simulink model "cst_robotarm_breach"  (R2020a)
settings: Solver=ode23t  StartTime=0.0  StopTime=40  FixedStep=0.0001  MaxStep=0.05  RelTol=1e-3  EnableMultiTasking=on
model workspace (MAT data in the model file):
  DCMotor_J = 0.0946866703633
  DCMotor_K = 0.477771340295
  DCMotor_Kf = 0.921434142151
  DCMotor_L = 0.000316454712175
  DCMotor_R = 4.99938152603
  Ts = 0.1
  dFilt = [1 -0.1202]
  nFilt = [0.4399 0.4399]
undefined symbols (not defined in the file or in its folder): X, Y, Z
libraries: sm_lib x244, fl_lib x75, nesl_utility x28, ee_lib x21
(part 5 of 6)

== system cst_robotarm_breach/6 DOF Robot Arm/6 DOF Robot Arm Mechanics/Forearm/ServoTJD_2_RIGID/servo_cover_2_RIGID ==
  ReferenceFrame : sm_lib/Frames and Transforms/Reference Frame
  Solid : sm_lib/Body Elements/File Solid  ExtGeomFileName=servo cover_Default_sldprt.STL  UnitType=Custom  ExtGeomFileUnits=mm  StepReaderType=HEX  ExportConvexHullGeometry=off  InertiaType=Custom  Mass=0.018198073455255783  MassUnits=kg  CenterOfMass=[19.173079671185903 9.8425000000000011 6.6069555093490839]  CenterOfMassUnits=mm  MomentsOfInertia=[1.0514460019053871 4.1870037592553642 4.7863110501402781]  MomentsOfInertiaUnits=kg*mm^2  ProductsOfInertia=[0 0.046415809435786888 0]  ProductsOfInertiaUnits=kg*mm^2  BasedOnType=Density  Density=1000  DensityUnits=kg/(m^3)  DoExposeReferenceFrame=on  SerializedFrames=<Frames/>  GraphicType=FromGeometry  MarkerShape=Sphere  MarkerSize=10  MarkerSizeUnits=m  GraphicVisPropType=SimpleVisualProperties  GraphicDiffuseColor=[0.6 0.6 0.6]  GraphicSpecularColor=[0.5 0.5 0.5 1.0]  GraphicAmbientColor=[0.15 0.15 0.15 1.0]  GraphicEmissiveColor=[0.0 0.0 0.0 1.0]  GraphicShininess=75  GraphicOpacity=1
  F : PMIOPort  Side=Left
  connections:
  Solid/RConn1 -- ReferenceFrame/RConn1 -- F/RConn1

== system cst_robotarm_breach/6 DOF Robot Arm/6 DOF Robot Arm Mechanics/Forearm/UpperArm_1_RIGID/BaseRef_1_RIGID ==
  ReferenceFrame : sm_lib/Frames and Transforms/Reference Frame
  Solid : sm_lib/Body Elements/File Solid  ExtGeomFileName=BaseRef_Default_sldprt.STL  UnitType=Custom  ExtGeomFileUnits=in  StepReaderType=HEX  ExportConvexHullGeometry=off  InertiaType=Custom  Mass=0.0048917083782427382  MassUnits=kg  CenterOfMass=[-1.7039170891361811e-10 0.2623949674376988 1.6125651751179532e-08]  CenterOfMassUnits=in  MomentsOfInertia=[0.0003243123013680548 0.00029766954875355879 0.00032242565061571212]  MomentsOfInertiaUnits=kg*in^2  ProductsOfInertia=[-6.4526471956204744e-12 2.3575705931561807e-11 0]  ProductsOfInertiaUnits=kg*in^2  BasedOnType=Density  Density=1000  DensityUnits=kg/(m^3)  DoExposeReferenceFrame=on  SerializedFrames=<Frames/>  GraphicType=FromGeometry  MarkerShape=Sphere  MarkerSize=10  MarkerSizeUnits=m  GraphicVisPropType=SimpleVisualProperties  GraphicDiffuseColor=[0.6 0.8 1.0]  GraphicSpecularColor=[0.5 0.5 0.5 1.0]  GraphicAmbientColor=[0.15 0.15 0.15 1.0]  GraphicEmissiveColor=[0.0 0.0 0.0 1.0]  GraphicShininess=75  GraphicOpacity=1
  F : PMIOPort  Side=Left
  connections:
  Solid/RConn1 -- ReferenceFrame/RConn1 -- F/RConn1

== system cst_robotarm_breach/6 DOF Robot Arm/6 DOF Robot Arm Mechanics/Forearm/UpperArm_1_RIGID/BaseRef_2_RIGID ==
  ReferenceFrame : sm_lib/Frames and Transforms/Reference Frame
  Solid : sm_lib/Body Elements/File Solid  ExtGeomFileName=BaseRef_Default_sldprt.STL  UnitType=Custom  ExtGeomFileUnits=in  StepReaderType=HEX  ExportConvexHullGeometry=off  InertiaType=Custom  Mass=0.0048917083782427382  MassUnits=kg  CenterOfMass=[-1.7039170891361811e-10 0.2623949674376988 1.6125651751179532e-08]  CenterOfMassUnits=in  MomentsOfInertia=[0.0003243123013680548 0.00029766954875355879 0.00032242565061571212]  MomentsOfInertiaUnits=kg*in^2  ProductsOfInertia=[-6.4526471956204744e-12 2.3575705931561807e-11 0]  ProductsOfInertiaUnits=kg*in^2  BasedOnType=Density  Density=1000  DensityUnits=kg/(m^3)  DoExposeReferenceFrame=on  SerializedFrames=<Frames/>  GraphicType=FromGeometry  MarkerShape=Sphere  MarkerSize=10  MarkerSizeUnits=m  GraphicVisPropType=SimpleVisualProperties  GraphicDiffuseColor=[0.6 0.8 1.0]  GraphicSpecularColor=[0.5 0.5 0.5 1.0]  GraphicAmbientColor=[0.15 0.15 0.15 1.0]  GraphicEmissiveColor=[0.0 0.0 0.0 1.0]  GraphicShininess=75  GraphicOpacity=1
  F : PMIOPort  Side=Left
  connections:
  Solid/RConn1 -- ReferenceFrame/RConn1 -- F/RConn1

== system cst_robotarm_breach/6 DOF Robot Arm/6 DOF Robot Arm Mechanics/Forearm/UpperArm_1_RIGID/asb_04_1_RIGID ==
  ReferenceFrame : sm_lib/Frames and Transforms/Reference Frame
  Solid : sm_lib/Body Elements/File Solid  ExtGeomFileName=asb-04_Default_sldprt.STL  UnitType=Custom  ExtGeomFileUnits=mm  StepReaderType=HEX  ExportConvexHullGeometry=off  InertiaType=Custom  Mass=0.012502145661798053  MassUnits=kg  CenterOfMass=[0 6.0244491918420078 4.4962453719208186]  CenterOfMassUnits=mm  MomentsOfInertia=[2.428586923331026 4.8465793426778037 3.7918219462476519]  MomentsOfInertiaUnits=kg*mm^2  ProductsOfInertia=[-0.330066861743673 0 0]  ProductsOfInertiaUnits=kg*mm^2  BasedOnType=Density  Density=1000  DensityUnits=kg/(m^3)  DoExposeReferenceFrame=on  SerializedFrames=<Frames/>  GraphicType=FromGeometry  MarkerShape=Sphere  MarkerSize=10  MarkerSizeUnits=m  GraphicVisPropType=SimpleVisualProperties  GraphicDiffuseColor=[0.6 0.8 1.0]  GraphicSpecularColor=[0.5 0.5 0.5 1.0]  GraphicAmbientColor=[0.15 0.15 0.15 1.0]  GraphicEmissiveColor=[0.0 0.0 0.0 1.0]  GraphicShininess=75  GraphicOpacity=1
  F : PMIOPort  Side=Left
  connections:
  Solid/RConn1 -- ReferenceFrame/RConn1 -- F/RConn1

== system cst_robotarm_breach/6 DOF Robot Arm/6 DOF Robot Arm Mechanics/Forearm/UpperArm_1_RIGID/asb_04_2_RIGID ==
  ReferenceFrame : sm_lib/Frames and Transforms/Reference Frame
  Solid : sm_lib/Body Elements/File Solid  ExtGeomFileName=asb-04_Default_sldprt.STL  UnitType=Custom  ExtGeomFileUnits=mm  StepReaderType=HEX  ExportConvexHullGeometry=off  InertiaType=Custom  Mass=0.012502145661798053  MassUnits=kg  CenterOfMass=[0 6.0244491918420078 4.4962453719208186]  CenterOfMassUnits=mm  MomentsOfInertia=[2.428586923331026 4.8465793426778037 3.7918219462476519]  MomentsOfInertiaUnits=kg*mm^2  ProductsOfInertia=[-0.330066861743673 0 0]  ProductsOfInertiaUnits=kg*mm^2  BasedOnType=Density  Density=1000  DensityUnits=kg/(m^3)  DoExposeReferenceFrame=on  SerializedFrames=<Frames/>  GraphicType=FromGeometry  MarkerShape=Sphere  MarkerSize=10  MarkerSizeUnits=m  GraphicVisPropType=SimpleVisualProperties  GraphicDiffuseColor=[0.6 0.8 1.0]  GraphicSpecularColor=[0.5 0.5 0.5 1.0]  GraphicAmbientColor=[0.15 0.15 0.15 1.0]  GraphicEmissiveColor=[0.0 0.0 0.0 1.0]  GraphicShininess=75  GraphicOpacity=1
  F : PMIOPort  Side=Left
  connections:
  Solid/RConn1 -- ReferenceFrame/RConn1 -- F/RConn1

== system cst_robotarm_breach/6 DOF Robot Arm/6 DOF Robot Arm Mechanics/Forearm/UpperArm_1_RIGID/asb_06_1_RIGID ==
  ReferenceFrame : sm_lib/Frames and Transforms/Reference Frame
  Solid : sm_lib/Body Elements/File Solid  ExtGeomFileName=asb-06_Default_sldprt.STL  UnitType=Custom  ExtGeomFileUnits=mm  StepReaderType=HEX  ExportConvexHullGeometry=off  InertiaType=Custom  Mass=0.0080717858989095559  MassUnits=kg  CenterOfMass=[-9.9260131397596147 6.2234969189440275 0]  CenterOfMassUnits=mm  MomentsOfInertia=[0.871366295206629 1.2650443449488296 1.3334610494978376]  MomentsOfInertiaUnits=kg*mm^2  ProductsOfInertia=[0 0 -0.36019818264401821]  ProductsOfInertiaUnits=kg*mm^2  BasedOnType=Density  Density=1000  DensityUnits=kg/(m^3)  DoExposeReferenceFrame=on  SerializedFrames=<Frames/>  GraphicType=FromGeometry  MarkerShape=Sphere  MarkerSize=10  MarkerSizeUnits=m  GraphicVisPropType=SimpleVisualProperties  GraphicDiffuseColor=[0.6 0.8 1.0]  GraphicSpecularColor=[0.5 0.5 0.5 1.0]  GraphicAmbientColor=[0.15 0.15 0.15 1.0]  GraphicEmissiveColor=[0.0 0.0 0.0 1.0]  GraphicShininess=75  GraphicOpacity=1
  F : PMIOPort  Side=Left
  connections:
  Solid/RConn1 -- ReferenceFrame/RConn1 -- F/RConn1

== system cst_robotarm_breach/6 DOF Robot Arm/6 DOF Robot Arm Mechanics/Forearm/UpperArm_1_RIGID/asb_06_2_RIGID ==
  ReferenceFrame : sm_lib/Frames and Transforms/Reference Frame
  Solid : sm_lib/Body Elements/File Solid  ExtGeomFileName=asb-06_Default_sldprt.STL  UnitType=Custom  ExtGeomFileUnits=mm  StepReaderType=HEX  ExportConvexHullGeometry=off  InertiaType=Custom  Mass=0.0080717858989095559  MassUnits=kg  CenterOfMass=[-9.9260131397596147 6.2234969189440275 0]  CenterOfMassUnits=mm  MomentsOfInertia=[0.871366295206629 1.2650443449488296 1.3334610494978376]  MomentsOfInertiaUnits=kg*mm^2  ProductsOfInertia=[0 0 -0.36019818264401821]  ProductsOfInertiaUnits=kg*mm^2  BasedOnType=Density  Density=1000  DensityUnits=kg/(m^3)  DoExposeReferenceFrame=on  SerializedFrames=<Frames/>  GraphicType=FromGeometry  MarkerShape=Sphere  MarkerSize=10  MarkerSizeUnits=m  GraphicVisPropType=SimpleVisualProperties  GraphicDiffuseColor=[0.6 0.8 1.0]  GraphicSpecularColor=[0.5 0.5 0.5 1.0]  GraphicAmbientColor=[0.15 0.15 0.15 1.0]  GraphicEmissiveColor=[0.0 0.0 0.0 1.0]  GraphicShininess=75  GraphicOpacity=1
  F : PMIOPort  Side=Left
  connections:
  Solid/RConn1 -- ReferenceFrame/RConn1 -- F/RConn1

== system cst_robotarm_breach/6 DOF Robot Arm/6 DOF Robot Arm Mechanics/Forearm/UpperArm_1_RIGID/at_06_1_RIGID ==
  ReferenceFrame : sm_lib/Frames and Transforms/Reference Frame
  Solid : sm_lib/Body Elements/File Solid  ExtGeomFileName=at-06_Default_sldprt.STL  UnitType=Custom  ExtGeomFileUnits=mm  StepReaderType=HEX  ExportConvexHullGeometry=off  InertiaType=Custom  Mass=0.0081837500372110746  MassUnits=kg  CenterOfMass=[-1.816422467996463e-08 -5.0466522298709023e-07 42.862382459231029]  CenterOfMassUnits=mm  MomentsOfInertia=[5.0863463702079237 5.0907330809753244 0.28704603607760404]  MomentsOfInertiaUnits=kg*mm^2  ProductsOfInertia=[2.9075703783527806e-06 -7.690574725829705e-07 -3.4008607477439507e-06]  ProductsOfInertiaUnits=kg*mm^2  BasedOnType=Density  Density=1000  DensityUnits=kg/(m^3)  DoExposeReferenceFrame=on  SerializedFrames=<Frames/>  GraphicType=FromGeometry  MarkerShape=Sphere  MarkerSize=10  MarkerSizeUnits=m  GraphicVisPropType=SimpleVisualProperties  GraphicDiffuseColor=[0.6 0.8 1.0]  GraphicSpecularColor=[0.5 0.5 0.5 1.0]  GraphicAmbientColor=[0.15 0.15 0.15 1.0]  GraphicEmissiveColor=[0.0 0.0 0.0 1.0]  GraphicShininess=75  GraphicOpacity=1
  F : PMIOPort  Side=Left
  connections:
  Solid/RConn1 -- ReferenceFrame/RConn1 -- F/RConn1

== system cst_robotarm_breach/6 DOF Robot Arm/6 DOF Robot Arm Mechanics/Gripper/LeftGripper_1_RIGID/GripperLeft_1_RIGID ==
  ReferenceFrame : sm_lib/Frames and Transforms/Reference Frame
  Solid : sm_lib/Body Elements/File Solid  ExtGeomFileName=GripperLeft_Default_sldprt.STL  UnitType=Custom  ExtGeomFileUnits=mm  StepReaderType=HEX  ExportConvexHullGeometry=off  InertiaType=Custom  Mass=0.0054837472367652322  MassUnits=kg  CenterOfMass=[7.5312895024124931 -5.3079249665701553 1.2060569262790406]  CenterOfMassUnits=mm  MomentsOfInertia=[0.28663713454900869 0.89920807040371731 0.71744303970434065]  MomentsOfInertiaUnits=kg*mm^2  ProductsOfInertia=[-0.013166116487360812 0.10888352596311582 0.088149803089705936]  ProductsOfInertiaUnits=kg*mm^2  BasedOnType=Density  Density=1000  DensityUnits=kg/(m^3)  DoExposeReferenceFrame=on  SerializedFrames=<Frames/>  GraphicType=FromGeometry  MarkerShape=Sphere  MarkerSize=10  MarkerSizeUnits=m  GraphicVisPropType=SimpleVisualProperties  GraphicDiffuseColor=[0.4 0.4 0.4]  GraphicSpecularColor=[0.5 0.5 0.5 1.0]  GraphicAmbientColor=[0.15 0.15 0.15 1.0]  GraphicEmissiveColor=[0.0 0.0 0.0 1.0]  GraphicShininess=75  GraphicOpacity=1
  F : PMIOPort  Side=Left
  connections:
  Solid/RConn1 -- ReferenceFrame/RConn1 -- F/RConn1

== system cst_robotarm_breach/6 DOF Robot Arm/6 DOF Robot Arm Mechanics/Gripper/LeftGripper_1_RIGID/gripperPad_1_RIGID ==
  ReferenceFrame : sm_lib/Frames and Transforms/Reference Frame
  Solid : sm_lib/Body Elements/File Solid  ExtGeomFileName=gripperPad_Default_sldprt.STL  UnitType=Custom  ExtGeomFileUnits=mm  StepReaderType=HEX  ExportConvexHullGeometry=off  InertiaType=Custom  Mass=0.0014400000000000001  MassUnits=kg  CenterOfMass=[0 0 0]  CenterOfMassUnits=mm  MomentsOfInertia=[0.040799999999999996 0.049920000000000006 0.086880000000000027]  MomentsOfInertiaUnits=kg*mm^2  ProductsOfInertia=[0 0 0]  ProductsOfInertiaUnits=kg*mm^2  BasedOnType=Density  Density=1000  DensityUnits=kg/(m^3)  DoExposeReferenceFrame=on  SerializedFrames=<Frames/>  GraphicType=FromGeometry  MarkerShape=Sphere  MarkerSize=10  MarkerSizeUnits=m  GraphicVisPropType=SimpleVisualProperties  GraphicDiffuseColor=[0.3 0.3 0.3]  GraphicSpecularColor=[0.5 0.5 0.5 1.0]  GraphicAmbientColor=[0.15 0.15 0.15 1.0]  GraphicEmissiveColor=[0.0 0.0 0.0 1.0]  GraphicShininess=75  GraphicOpacity=1
  F : PMIOPort  Side=Left
  connections:
  Solid/RConn1 -- ReferenceFrame/RConn1 -- F/RConn1

== system cst_robotarm_breach/6 DOF Robot Arm/6 DOF Robot Arm Mechanics/Gripper/RightGripper_1_RIGID/GripperRight_1_RIGID ==
  ReferenceFrame : sm_lib/Frames and Transforms/Reference Frame
  Solid : sm_lib/Body Elements/File Solid  ExtGeomFileName=GripperRight_Default_sldprt.STL  UnitType=Custom  ExtGeomFileUnits=mm  StepReaderType=HEX  ExportConvexHullGeometry=off  InertiaType=Custom  Mass=0.0054837472367652304  MassUnits=kg  CenterOfMass=[7.5312895024124948 -5.3079249665701571 -1.2060569262790404]  CenterOfMassUnits=mm  MomentsOfInertia=[0.28663713454900847 0.8992080704037172 0.71744303970434065]  MomentsOfInertiaUnits=kg*mm^2  ProductsOfInertia=[0.013166116487360839 -0.10888352596311589 0.088149803089706033]  ProductsOfInertiaUnits=kg*mm^2  BasedOnType=Density  Density=1000  DensityUnits=kg/(m^3)  DoExposeReferenceFrame=on  SerializedFrames=<Frames/>  GraphicType=FromGeometry  MarkerShape=Sphere  MarkerSize=10  MarkerSizeUnits=m  GraphicVisPropType=SimpleVisualProperties  GraphicDiffuseColor=[0.4 0.4 0.4]  GraphicSpecularColor=[0.5 0.5 0.5 1.0]  GraphicAmbientColor=[0.15 0.15 0.15 1.0]  GraphicEmissiveColor=[0.0 0.0 0.0 1.0]  GraphicShininess=75  GraphicOpacity=1
  F : PMIOPort  Side=Left
  connections:
  Solid/RConn1 -- ReferenceFrame/RConn1 -- F/RConn1

== system cst_robotarm_breach/6 DOF Robot Arm/6 DOF Robot Arm Mechanics/Gripper/RightGripper_1_RIGID/gripperPad_1_RIGID ==
  ReferenceFrame : sm_lib/Frames and Transforms/Reference Frame
  Solid : sm_lib/Body Elements/File Solid  ExtGeomFileName=gripperPad_Default_sldprt.STL  UnitType=Custom  ExtGeomFileUnits=mm  StepReaderType=HEX  ExportConvexHullGeometry=off  InertiaType=Custom  Mass=0.0014400000000000001  MassUnits=kg  CenterOfMass=[0 0 0]  CenterOfMassUnits=mm  MomentsOfInertia=[0.040799999999999996 0.049920000000000006 0.086880000000000027]  MomentsOfInertiaUnits=kg*mm^2  ProductsOfInertia=[0 0 0]  ProductsOfInertiaUnits=kg*mm^2  BasedOnType=Density  Density=1000  DensityUnits=kg/(m^3)  DoExposeReferenceFrame=on  SerializedFrames=<Frames/>  GraphicType=FromGeometry  MarkerShape=Sphere  MarkerSize=10  MarkerSizeUnits=m  GraphicVisPropType=SimpleVisualProperties  GraphicDiffuseColor=[0.3 0.3 0.3]  GraphicSpecularColor=[0.5 0.5 0.5 1.0]  GraphicAmbientColor=[0.15 0.15 0.15 1.0]  GraphicEmissiveColor=[0.0 0.0 0.0 1.0]  GraphicShininess=75  GraphicOpacity=1
  F : PMIOPort  Side=Left
  connections:
  Solid/RConn1 -- ReferenceFrame/RConn1 -- F/RConn1

== system cst_robotarm_breach/6 DOF Robot Arm/6 DOF Robot Arm Mechanics/Hand/ServoTJD2_1_RIGID/bottom_cover_1_RIGID ==
  ReferenceFrame : sm_lib/Frames and Transforms/Reference Frame
  Solid : sm_lib/Body Elements/File Solid  ExtGeomFileName=bottom cover_Default_sldprt.STL  UnitType=Custom  ExtGeomFileUnits=mm  StepReaderType=HEX  ExportConvexHullGeometry=off  InertiaType=Custom  Mass=0.0069725116500885713  MassUnits=kg  CenterOfMass=[0 0.85958385692466177 0]  CenterOfMassUnits=mm  MomentsOfInertia=[0.21879995145338263 1.0303249150901777 0.81533794134290127]  MomentsOfInertiaUnits=kg*mm^2  ProductsOfInertia=[0 0 0]  ProductsOfInertiaUnits=kg*mm^2  BasedOnType=Density  Density=1000  DensityUnits=kg/(m^3)  DoExposeReferenceFrame=on  SerializedFrames=<Frames/>  GraphicType=FromGeometry  MarkerShape=Sphere  MarkerSize=10  MarkerSizeUnits=m  GraphicVisPropType=SimpleVisualProperties  GraphicDiffuseColor=[0.4 0.4 0.4]  GraphicSpecularColor=[0.5 0.5 0.5 1.0]  GraphicAmbientColor=[0.15 0.15 0.15 1.0]  GraphicEmissiveColor=[0.0 0.0 0.0 1.0]  GraphicShininess=75  GraphicOpacity=1
  F : PMIOPort  Side=Left
  connections:
  Solid/RConn1 -- ReferenceFrame/RConn1 -- F/RConn1

== system cst_robotarm_breach/6 DOF Robot Arm/6 DOF Robot Arm Mechanics/Hand/ServoTJD2_1_RIGID/servo_Case_1_RIGID ==
  ReferenceFrame : sm_lib/Frames and Transforms/Reference Frame
  Solid : sm_lib/Body Elements/File Solid  ExtGeomFileName=servo Case_Default_sldprt.STL  UnitType=Custom  ExtGeomFileUnits=mm  StepReaderType=HEX  ExportConvexHullGeometry=off  InertiaType=Custom  Mass=0.024788567791665928  MassUnits=kg  CenterOfMass=[0.08042125391634411 -6.0857711413150408 -0.045303315504018803]  CenterOfMassUnits=mm  MomentsOfInertia=[2.4475554038950817 5.416405903149534 5.3480430794560796]  MomentsOfInertiaUnits=kg*mm^2  ProductsOfInertia=[0.0035757453477574665 0.0080258931443943603 -0.048088274914116991]  ProductsOfInertiaUnits=kg*mm^2  BasedOnType=Density  Density=1000  DensityUnits=kg/(m^3)  DoExposeReferenceFrame=on  SerializedFrames=<Frames/>  GraphicType=FromGeometry  MarkerShape=Sphere  MarkerSize=10  MarkerSizeUnits=m  GraphicVisPropType=SimpleVisualProperties  GraphicDiffuseColor=[0.4 0.4 0.4]  GraphicSpecularColor=[0.5 0.5 0.5 1.0]  GraphicAmbientColor=[0.15 0.15 0.15 1.0]  GraphicEmissiveColor=[0.0 0.0 0.0 1.0]  GraphicShininess=75  GraphicOpacity=1
  F : PMIOPort  Side=Left
  connections:
  Solid/RConn1 -- ReferenceFrame/RConn1 -- F/RConn1

== system cst_robotarm_breach/6 DOF Robot Arm/6 DOF Robot Arm Mechanics/Hand/ServoTJD2_1_RIGID/servo_cover_2_RIGID ==
  ReferenceFrame : sm_lib/Frames and Transforms/Reference Frame
  Solid : sm_lib/Body Elements/File Solid  ExtGeomFileName=servo cover_Default_sldprt.STL  UnitType=Custom  ExtGeomFileUnits=mm  StepReaderType=HEX  ExportConvexHullGeometry=off  InertiaType=Custom  Mass=0.018198073455255783  MassUnits=kg  CenterOfMass=[19.173079671185903 9.8425000000000011 6.6069555093490839]  CenterOfMassUnits=mm  MomentsOfInertia=[1.0514460019053871 4.1870037592553642 4.7863110501402781]  MomentsOfInertiaUnits=kg*mm^2  ProductsOfInertia=[0 0.046415809435786888 0]  ProductsOfInertiaUnits=kg*mm^2  BasedOnType=Density  Density=1000  DensityUnits=kg/(m^3)  DoExposeReferenceFrame=on  SerializedFrames=<Frames/>  GraphicType=FromGeometry  MarkerShape=Sphere  MarkerSize=10  MarkerSizeUnits=m  GraphicVisPropType=SimpleVisualProperties  GraphicDiffuseColor=[0.6 0.6 0.6]  GraphicSpecularColor=[0.5 0.5 0.5 1.0]  GraphicAmbientColor=[0.15 0.15 0.15 1.0]  GraphicEmissiveColor=[0.0 0.0 0.0 1.0]  GraphicShininess=75  GraphicOpacity=1
  F : PMIOPort  Side=Left
  connections:
  Solid/RConn1 -- ReferenceFrame/RConn1 -- F/RConn1

== system cst_robotarm_breach/6 DOF Robot Arm/6 DOF Robot Arm Mechanics/Turntable/ServoTJD_1_RIGID/ServoHornPlastic_1_RIGID ==
  ReferenceFrame : sm_lib/Frames and Transforms/Reference Frame
  Solid : sm_lib/Body Elements/File Solid  ExtGeomFileName=ServoHornPlastic_Default_sldprt.STL  UnitType=Custom  ExtGeomFileUnits=mm  StepReaderType=HEX  ExportConvexHullGeometry=off  InertiaType=Custom  Mass=0.0010704340009196711  MassUnits=kg  CenterOfMass=[0 -1.2011682426591921 0]  CenterOfMassUnits=mm  MomentsOfInertia=[0.037722424473240444 0.072621190507680802 0.036596357544803754]  MomentsOfInertiaUnits=kg*mm^2  ProductsOfInertia=[0 0 0]  ProductsOfInertiaUnits=kg*mm^2  BasedOnType=Density  Density=1000  DensityUnits=kg/(m^3)  DoExposeReferenceFrame=on  SerializedFrames=<Frames/>  GraphicType=FromGeometry  MarkerShape=Sphere  MarkerSize=10  MarkerSizeUnits=m  GraphicVisPropType=SimpleVisualProperties  GraphicDiffuseColor=[1.0 1.0 1.0]  GraphicSpecularColor=[0.5 0.5 0.5 1.0]  GraphicAmbientColor=[0.15 0.15 0.15 1.0]  GraphicEmissiveColor=[0.0 0.0 0.0 1.0]  GraphicShininess=75  GraphicOpacity=1
  F : PMIOPort  Side=Left
  connections:
  Solid/RConn1 -- ReferenceFrame/RConn1 -- F/RConn1

== system cst_robotarm_breach/6 DOF Robot Arm/6 DOF Robot Arm Mechanics/Turntable/ServoTJD_1_RIGID/bottom_cover_1_RIGID ==
  ReferenceFrame : sm_lib/Frames and Transforms/Reference Frame
  Solid : sm_lib/Body Elements/File Solid  ExtGeomFileName=bottom cover_Default_sldprt.STL  UnitType=Custom  ExtGeomFileUnits=mm  StepReaderType=HEX  ExportConvexHullGeometry=off  InertiaType=Custom  Mass=0.0069725116500885713  MassUnits=kg  CenterOfMass=[0 0.85958385692466177 0]  CenterOfMassUnits=mm  MomentsOfInertia=[0.21879995145338263 1.0303249150901777 0.81533794134290127]  MomentsOfInertiaUnits=kg*mm^2  ProductsOfInertia=[0 0 0]  ProductsOfInertiaUnits=kg*mm^2  BasedOnType=Density  Density=1000  DensityUnits=kg/(m^3)  DoExposeReferenceFrame=on  SerializedFrames=<Frames/>  GraphicType=FromGeometry  MarkerShape=Sphere  MarkerSize=10  MarkerSizeUnits=m  GraphicVisPropType=SimpleVisualProperties  GraphicDiffuseColor=[0.4 0.4 0.4]  GraphicSpecularColor=[0.5 0.5 0.5 1.0]  GraphicAmbientColor=[0.15 0.15 0.15 1.0]  GraphicEmissiveColor=[0.0 0.0 0.0 1.0]  GraphicShininess=75  GraphicOpacity=1
  F : PMIOPort  Side=Left
  connections:
  Solid/RConn1 -- ReferenceFrame/RConn1 -- F/RConn1

== system cst_robotarm_breach/6 DOF Robot Arm/6 DOF Robot Arm Mechanics/Turntable/ServoTJD_1_RIGID/servo_Case_1_RIGID ==
  ReferenceFrame : sm_lib/Frames and Transforms/Reference Frame
  Solid : sm_lib/Body Elements/File Solid  ExtGeomFileName=servo Case_Default_sldprt.STL  UnitType=Custom  ExtGeomFileUnits=mm  StepReaderType=HEX  ExportConvexHullGeometry=off  InertiaType=Custom  Mass=0.024788567791665928  MassUnits=kg  CenterOfMass=[0.08042125391634411 -6.0857711413150408 -0.045303315504018803]  CenterOfMassUnits=mm  MomentsOfInertia=[2.4475554038950817 5.416405903149534 5.3480430794560796]  MomentsOfInertiaUnits=kg*mm^2  ProductsOfInertia=[0.0035757453477574665 0.0080258931443943603 -0.048088274914116991]  ProductsOfInertiaUnits=kg*mm^2  BasedOnType=Density  Density=1000  DensityUnits=kg/(m^3)  DoExposeReferenceFrame=on  SerializedFrames=<Frames/>  GraphicType=FromGeometry  MarkerShape=Sphere  MarkerSize=10  MarkerSizeUnits=m  GraphicVisPropType=SimpleVisualProperties  GraphicDiffuseColor=[0.4 0.4 0.4]  GraphicSpecularColor=[0.5 0.5 0.5 1.0]  GraphicAmbientColor=[0.15 0.15 0.15 1.0]  GraphicEmissiveColor=[0.0 0.0 0.0 1.0]  GraphicShininess=75  GraphicOpacity=1
  F : PMIOPort  Side=Left
  connections:
  Solid/RConn1 -- ReferenceFrame/RConn1 -- F/RConn1

== system cst_robotarm_breach/6 DOF Robot Arm/6 DOF Robot Arm Mechanics/Turntable/ServoTJD_1_RIGID/servo_cover_2_RIGID ==
  ReferenceFrame : sm_lib/Frames and Transforms/Reference Frame
  Solid : sm_lib/Body Elements/File Solid  ExtGeomFileName=servo cover_Default_sldprt.STL  UnitType=Custom  ExtGeomFileUnits=mm  StepReaderType=HEX  ExportConvexHullGeometry=off  InertiaType=Custom  Mass=0.018198073455255783  MassUnits=kg  CenterOfMass=[19.173079671185903 9.8425000000000011 6.6069555093490839]  CenterOfMassUnits=mm  MomentsOfInertia=[1.0514460019053871 4.1870037592553642 4.7863110501402781]  MomentsOfInertiaUnits=kg*mm^2  ProductsOfInertia=[0 0.046415809435786888 0]  ProductsOfInertiaUnits=kg*mm^2  BasedOnType=Density  Density=1000  DensityUnits=kg/(m^3)  DoExposeReferenceFrame=on  SerializedFrames=<Frames/>  GraphicType=FromGeometry  MarkerShape=Sphere  MarkerSize=10  MarkerSizeUnits=m  GraphicVisPropType=SimpleVisualProperties  GraphicDiffuseColor=[0.6 0.6 0.6]  GraphicSpecularColor=[0.5 0.5 0.5 1.0]  GraphicAmbientColor=[0.15 0.15 0.15 1.0]  GraphicEmissiveColor=[0.0 0.0 0.0 1.0]  GraphicShininess=75  GraphicOpacity=1
  F : PMIOPort  Side=Left
  connections:
  Solid/RConn1 -- ReferenceFrame/RConn1 -- F/RConn1

== system cst_robotarm_breach/6 DOF Robot Arm/6 DOF Robot Arm Mechanics/Turntable/ServoTJD_2_RIGID/ServoHornPlastic_1_RIGID ==
  ReferenceFrame : sm_lib/Frames and Transforms/Reference Frame
  Solid : sm_lib/Body Elements/File Solid  ExtGeomFileName=ServoHornPlastic_Default_sldprt.STL  UnitType=Custom  ExtGeomFileUnits=mm  StepReaderType=HEX  ExportConvexHullGeometry=off  InertiaType=Custom  Mass=0.0010704340009196711  MassUnits=kg  CenterOfMass=[0 -1.2011682426591921 0]  CenterOfMassUnits=mm  MomentsOfInertia=[0.037722424473240444 0.072621190507680802 0.036596357544803754]  MomentsOfInertiaUnits=kg*mm^2  ProductsOfInertia=[0 0 0]  ProductsOfInertiaUnits=kg*mm^2  BasedOnType=Density  Density=1000  DensityUnits=kg/(m^3)  DoExposeReferenceFrame=on  SerializedFrames=<Frames/>  GraphicType=FromGeometry  MarkerShape=Sphere  MarkerSize=10  MarkerSizeUnits=m  GraphicVisPropType=SimpleVisualProperties  GraphicDiffuseColor=[1.0 1.0 1.0]  GraphicSpecularColor=[0.5 0.5 0.5 1.0]  GraphicAmbientColor=[0.15 0.15 0.15 1.0]  GraphicEmissiveColor=[0.0 0.0 0.0 1.0]  GraphicShininess=75  GraphicOpacity=1
  F : PMIOPort  Side=Left
  connections:
  Solid/RConn1 -- ReferenceFrame/RConn1 -- F/RConn1

== system cst_robotarm_breach/6 DOF Robot Arm/6 DOF Robot Arm Mechanics/Turntable/ServoTJD_2_RIGID/bottom_cover_1_RIGID ==
  ReferenceFrame : sm_lib/Frames and Transforms/Reference Frame
  Solid : sm_lib/Body Elements/File Solid  ExtGeomFileName=bottomCover_Default_sldprt.STL  UnitType=Custom  ExtGeomFileUnits=mm  StepReaderType=HEX  ExportConvexHullGeometry=off  InertiaType=Custom  Mass=0.0069725116500885713  MassUnits=kg  CenterOfMass=[0 0.85958385692466177 0]  CenterOfMassUnits=mm  MomentsOfInertia=[0.21879995145338263 1.0303249150901777 0.81533794134290127]  MomentsOfInertiaUnits=kg*mm^2  ProductsOfInertia=[0 0 0]  ProductsOfInertiaUnits=kg*mm^2  BasedOnType=Density  Density=1000  DensityUnits=kg/(m^3)  DoExposeReferenceFrame=on  SerializedFrames=<Frames/>  GraphicType=FromGeometry  MarkerShape=Sphere  MarkerSize=10  MarkerSizeUnits=m  GraphicVisPropType=SimpleVisualProperties  GraphicDiffuseColor=[0.4 0.4 0.4]  GraphicSpecularColor=[0.5 0.5 0.5 1.0]  GraphicAmbientColor=[0.15 0.15 0.15 1.0]  GraphicEmissiveColor=[0.0 0.0 0.0 1.0]  GraphicShininess=75  GraphicOpacity=1
  F : PMIOPort  Side=Left
  connections:
  Solid/RConn1 -- ReferenceFrame/RConn1 -- F/RConn1

== system cst_robotarm_breach/6 DOF Robot Arm/6 DOF Robot Arm Mechanics/Turntable/ServoTJD_2_RIGID/servo_Case_1_RIGID ==
  ReferenceFrame : sm_lib/Frames and Transforms/Reference Frame
  Solid : sm_lib/Body Elements/File Solid  ExtGeomFileName=servoCase_Default_sldprt.STL  UnitType=Custom  ExtGeomFileUnits=mm  StepReaderType=HEX  ExportConvexHullGeometry=off  InertiaType=Custom  Mass=0.024788567791665928  MassUnits=kg  CenterOfMass=[0.08042125391634411 -6.0857711413150408 -0.045303315504018803]  CenterOfMassUnits=mm  MomentsOfInertia=[2.4475554038950817 5.416405903149534 5.3480430794560796]  MomentsOfInertiaUnits=kg*mm^2  ProductsOfInertia=[0.0035757453477574665 0.0080258931443943603 -0.048088274914116991]  ProductsOfInertiaUnits=kg*mm^2  BasedOnType=Density  Density=1000  DensityUnits=kg/(m^3)  DoExposeReferenceFrame=on  SerializedFrames=<Frames/>  GraphicType=FromGeometry  MarkerShape=Sphere  MarkerSize=10  MarkerSizeUnits=m  GraphicVisPropType=SimpleVisualProperties  GraphicDiffuseColor=[0.4 0.4 0.4]  GraphicSpecularColor=[0.5 0.5 0.5 1.0]  GraphicAmbientColor=[0.15 0.15 0.15 1.0]  GraphicEmissiveColor=[0.0 0.0 0.0 1.0]  GraphicShininess=75  GraphicOpacity=1
  F : PMIOPort  Side=Left
  connections:
  Solid/RConn1 -- ReferenceFrame/RConn1 -- F/RConn1

== system cst_robotarm_breach/6 DOF Robot Arm/6 DOF Robot Arm Mechanics/Turntable/ServoTJD_2_RIGID/servo_cover_2_RIGID ==
  ReferenceFrame : sm_lib/Frames and Transforms/Reference Frame
  Solid : sm_lib/Body Elements/File Solid  ExtGeomFileName=servoCover_Default_sldprt.STL  UnitType=Custom  ExtGeomFileUnits=mm  StepReaderType=HEX  ExportConvexHullGeometry=off  InertiaType=Custom  Mass=0.018198073455255783  MassUnits=kg  CenterOfMass=[19.173079671185903 9.8425000000000011 6.6069555093490839]  CenterOfMassUnits=mm  MomentsOfInertia=[1.0514460019053871 4.1870037592553642 4.7863110501402781]  MomentsOfInertiaUnits=kg*mm^2  ProductsOfInertia=[0 0.046415809435786888 0]  ProductsOfInertiaUnits=kg*mm^2  BasedOnType=Density  Density=1000  DensityUnits=kg/(m^3)  DoExposeReferenceFrame=on  SerializedFrames=<Frames/>  GraphicType=FromGeometry  MarkerShape=Sphere  MarkerSize=10  MarkerSizeUnits=m  GraphicVisPropType=SimpleVisualProperties  GraphicDiffuseColor=[0.6 0.6 0.6]  GraphicSpecularColor=[0.5 0.5 0.5 1.0]  GraphicAmbientColor=[0.15 0.15 0.15 1.0]  GraphicEmissiveColor=[0.0 0.0 0.0 1.0]  GraphicShininess=75  GraphicOpacity=1
  F : PMIOPort  Side=Left
  connections:
  Solid/RConn1 -- ReferenceFrame/RConn1 -- F/RConn1

== system cst_robotarm_breach/6 DOF Robot Arm/6 DOF Robot Arm Mechanics/Wrist/MotorWristAsm_1_RIGID/BB_01_1_RIGID ==
  ReferenceFrame : sm_lib/Frames and Transforms/Reference Frame
  Solid : sm_lib/Body Elements/File Solid  ExtGeomFileName=BB-01_Default_sldprt.STL  UnitType=Custom  ExtGeomFileUnits=mm  StepReaderType=HEX  ExportConvexHullGeometry=off  InertiaType=Custom  Mass=0.0017209417261250333  MassUnits=kg  CenterOfMass=[0 0 1.9700000000000317]  CenterOfMassUnits=mm  MomentsOfInertia=[0.01462455138119856 0.014624551381198564 0.025628067763636773]  MomentsOfInertiaUnits=kg*mm^2  ProductsOfInertia=[0 0 0]  ProductsOfInertiaUnits=kg*mm^2  BasedOnType=Density  Density=1000  DensityUnits=kg/(m^3)  DoExposeReferenceFrame=on  SerializedFrames=<Frames/>  GraphicType=FromGeometry  MarkerShape=Sphere  MarkerSize=10  MarkerSizeUnits=m  GraphicVisPropType=SimpleVisualProperties  GraphicDiffuseColor=[0.8 1.0 0.6]  GraphicSpecularColor=[0.5 0.5 0.5 1.0]  GraphicAmbientColor=[0.15 0.15 0.15 1.0]  GraphicEmissiveColor=[0.0 0.0 0.0 1.0]  GraphicShininess=75  GraphicOpacity=1
  F : PMIOPort  Side=Left
  connections:
  Solid/RConn1 -- ReferenceFrame/RConn1 -- F/RConn1

== system cst_robotarm_breach/6 DOF Robot Arm/6 DOF Robot Arm Mechanics/Wrist/MotorWristAsm_1_RIGID/ServoTJD2_1_RIGID ==
  ReferenceFrame : sm_lib/Frames and Transforms/Reference Frame
  Transform : sm_lib/Frames and Transforms/Rigid Transform  TranslationMethod=None  TranslationStandardOffset=0  TranslationLengthUnit=m  TranslationStandardAxis=+Z  TranslationCartesianOffset=[0 0 0]  TranslationROffset=0  TranslationROffsetUnits=m  TranslationZOffset=0  TranslationZOffsetUnits=m  TranslationThetaOffset=0  TranslationThetaOffsetUnits=deg  RotationMethod=None  RotationAngleUnits=deg  RotationStandardAxis=+Z  RotationAngle=0.0  RotationArbitraryAxis=[0 0 1]  FollAlignAxisA=+X  BaseAlignAxisA=+Y  FollAlignAxisB=+Y  BaseAlignAxisB=+Z  RotationSequenceAxes=FollowerAxes  RotationSequence=XYX  RotationSequenceAngles=[0 0 0]  RotationSequenceAnglesUnits=deg  RotationMatrix=[1 0 0; 0 1 0; 0 0 1]
  Transform1 : sm_lib/Frames and Transforms/Rigid Transform  TranslationMethod=Cartesian  TranslationStandardOffset=0  TranslationLengthUnit=mm  TranslationStandardAxis=+Z  TranslationCartesianOffset=[19.367500000000003 9.8424999999999976 -1.1906250000000007]  TranslationROffset=0  TranslationROffsetUnits=m  TranslationZOffset=0  TranslationZOffsetUnits=m  TranslationThetaOffset=0  TranslationThetaOffsetUnits=deg  RotationMethod=ArbitraryAxis  RotationAngleUnits=rad  RotationStandardAxis=+Z  RotationAngle=3.1415926535897931  RotationArbitraryAxis=[5.8878457842161208e-17 -0.70710678118654746 -0.70710678118654757]  FollAlignAxisA=+X  BaseAlignAxisA=+Y  FollAlignAxisB=+Y  BaseAlignAxisB=+Z  RotationSequenceAxes=FollowerAxes  RotationSequence=XYX  RotationSequenceAngles=[0 0 0]  RotationSequenceAnglesUnits=deg  RotationMatrix=[1 0 0; 0 1 0; 0 0 1]
  Transform2 : sm_lib/Frames and Transforms/Rigid Transform  TranslationMethod=Cartesian  TranslationStandardOffset=0  TranslationLengthUnit=mm  TranslationStandardAxis=+Z  TranslationCartesianOffset=[19.367499999999986 9.8425000000000047 -23.812500000000014]  TranslationROffset=0  TranslationROffsetUnits=m  TranslationZOffset=0  TranslationZOffsetUnits=m  TranslationThetaOffset=0  TranslationThetaOffsetUnits=deg  RotationMethod=ArbitraryAxis  RotationAngleUnits=rad  RotationStandardAxis=+Z  RotationAngle=1.5707963267948968  RotationArbitraryAxis=[1 0 0]  FollAlignAxisA=+X  BaseAlignAxisA=+Y  FollAlignAxisB=+Y  BaseAlignAxisB=+Z  RotationSequenceAxes=FollowerAxes  RotationSequence=XYX  RotationSequenceAngles=[0 0 0]  RotationSequenceAnglesUnits=deg  RotationMatrix=[1 0 0; 0 1 0; 0 0 1]
  Transform3 : sm_lib/Frames and Transforms/Rigid Transform  TranslationMethod=None  TranslationStandardOffset=0  TranslationLengthUnit=m  TranslationStandardAxis=+Z  TranslationCartesianOffset=[0 0 0]  TranslationROffset=0  TranslationROffsetUnits=m  TranslationZOffset=0  TranslationZOffsetUnits=m  TranslationThetaOffset=0  TranslationThetaOffsetUnits=deg  RotationMethod=None  RotationAngleUnits=deg  RotationStandardAxis=+Z  RotationAngle=0.0  RotationArbitraryAxis=[0 0 1]  FollAlignAxisA=+X  BaseAlignAxisA=+Y  FollAlignAxisB=+Y  BaseAlignAxisB=+Z  RotationSequenceAxes=FollowerAxes  RotationSequence=XYX  RotationSequenceAngles=[0 0 0]  RotationSequenceAnglesUnits=deg  RotationMatrix=[1 0 0; 0 1 0; 0 0 1]
  bottom_cover_1_RIGID : Subsystem
  servo_Case_1_RIGID : Subsystem
  servo_cover_2_RIGID : Subsystem
  F : PMIOPort  Side=Left
  connections:
  Transform/RConn1 -- servo_cover_2_RIGID/LConn1
  Transform1/RConn1 -- servo_Case_1_RIGID/LConn1
  Transform2/RConn1 -- bottom_cover_1_RIGID/LConn1
  ReferenceFrame/RConn1 -- Transform/LConn1 -- Transform3/RConn1 -- Transform2/LConn1 -- Transform1/LConn1
  Transform3/LConn1 -- F/RConn1

== system cst_robotarm_breach/6 DOF Robot Arm/6 DOF Robot Arm Mechanics/Wrist/MotorWristAsm_1_RIGID/asb_14_2_RIGID ==
  ReferenceFrame : sm_lib/Frames and Transforms/Reference Frame
  Solid : sm_lib/Body Elements/File Solid  ExtGeomFileName=asb-14_Default_sldprt.STL  UnitType=Custom  ExtGeomFileUnits=mm  StepReaderType=HEX  ExportConvexHullGeometry=off  InertiaType=Custom  Mass=0.0064054482551768026  MassUnits=kg  CenterOfMass=[30.876489525338485 0.76200000000000001 -35.309520359734812]  CenterOfMassUnits=mm  MomentsOfInertia=[1.7721561381596698 3.2106248609194923 1.4409482461576086]  MomentsOfInertiaUnits=kg*mm^2  ProductsOfInertia=[0 0.40144502992031489 0]  ProductsOfInertiaUnits=kg*mm^2  BasedOnType=Density  Density=1000  DensityUnits=kg/(m^3)  DoExposeReferenceFrame=on  SerializedFrames=<Frames/>  GraphicType=FromGeometry  MarkerShape=Sphere  MarkerSize=10  MarkerSizeUnits=m  GraphicVisPropType=SimpleVisualProperties  GraphicDiffuseColor=[0.8 1.0 0.6]  GraphicSpecularColor=[0.5 0.5 0.5 1.0]  GraphicAmbientColor=[0.15 0.15 0.15 1.0]  GraphicEmissiveColor=[0.0 0.0 0.0 1.0]  GraphicShininess=75  GraphicOpacity=1
  F : PMIOPort  Side=Left
  connections:
  Solid/RConn1 -- ReferenceFrame/RConn1 -- F/RConn1

== system cst_robotarm_breach/6 DOF Robot Arm/DC Motors/Bicep Motor1/Power Amplifier/SL2Vbrk ==
  Signal : Inport
  Electrical Reference1 : fl_lib/Electrical/Electrical Elements/Electrical Reference
      settings: SourceProductBaseCode=MT,SS
  Simulink to Physical Signal1 : nesl_utility/Simulink-PS Converter  PhysicalDomain=network_engine_domain  SubClassName=ps_input  LeftPortType=input  RightPortType=output  PseudoPeriodic=off  Frequencies=[]  NoiseDistribution=none  NoiseParameters=[]  Unit=V  AffineConversion=off  FilteringAndDerivatives=zero  SimscapeFilterOrder=1  InputFilterTimeConstant=.001  UdotUserProvided=0
      settings: SourceProductBaseCode=MT,SS
  Voltage Source : fl_lib/Electrical/Electrical Sources/Controlled Voltage Source
      settings: SourceProductBaseCode=MT,SS
  Volts : PMIOPort  Tag=PMCPort  Side=Right
  wires:
  Signal/1 -> Simulink to Physical Signal1/1
  connections:
  Electrical Reference1/LConn1 -- Voltage Source/RConn2
  Simulink to Physical Signal1/RConn1 -- Voltage Source/RConn1
  Voltage Source/LConn1 -- Volts/RConn1

== system cst_robotarm_breach/6 DOF Robot Arm/DC Motors/Bicep Motor1/Power Amplifier/SL2Vduty ==
  Signal : Inport
  Electrical Reference1 : fl_lib/Electrical/Electrical Elements/Electrical Reference
      settings: SourceProductBaseCode=MT,SS
  Simulink to Physical Signal1 : nesl_utility/Simulink-PS Converter  PhysicalDomain=network_engine_domain  SubClassName=ps_input  LeftPortType=input  RightPortType=output  PseudoPeriodic=off  Frequencies=[]  NoiseDistribution=none  NoiseParameters=[]  Unit=V  AffineConversion=off  FilteringAndDerivatives=zero  SimscapeFilterOrder=1  InputFilterTimeConstant=.001  UdotUserProvided=0
      settings: SourceProductBaseCode=MT,SS
  Voltage Source : fl_lib/Electrical/Electrical Sources/Controlled Voltage Source
      settings: SourceProductBaseCode=MT,SS
  Volts : PMIOPort  Tag=PMCPort  Side=Right
  wires:
  Signal/1 -> Simulink to Physical Signal1/1
  connections:
  Electrical Reference1/LConn1 -- Voltage Source/RConn2
  Simulink to Physical Signal1/RConn1 -- Voltage Source/RConn1
  Voltage Source/LConn1 -- Volts/RConn1

== system cst_robotarm_breach/6 DOF Robot Arm/DC Motors/Bicep Motor1/Power Amplifier/SL2Vrev ==
  Signal : Inport
  Electrical Reference1 : fl_lib/Electrical/Electrical Elements/Electrical Reference
      settings: SourceProductBaseCode=MT,SS
  Simulink to Physical Signal1 : nesl_utility/Simulink-PS Converter  PhysicalDomain=network_engine_domain  SubClassName=ps_input  LeftPortType=input  RightPortType=output  PseudoPeriodic=off  Frequencies=[]  NoiseDistribution=none  NoiseParameters=[]  Unit=V  AffineConversion=off  FilteringAndDerivatives=zero  SimscapeFilterOrder=1  InputFilterTimeConstant=.001  UdotUserProvided=0
      settings: SourceProductBaseCode=MT,SS
  Voltage Source : fl_lib/Electrical/Electrical Sources/Controlled Voltage Source
      settings: SourceProductBaseCode=MT,SS
  Volts : PMIOPort  Tag=PMCPort  Side=Right
  wires:
  Signal/1 -> Simulink to Physical Signal1/1
  connections:
  Voltage Source/LConn1 -- Volts/RConn1
  Simulink to Physical Signal1/RConn1 -- Voltage Source/RConn1
  Electrical Reference1/LConn1 -- Voltage Source/RConn2

== system cst_robotarm_breach/6 DOF Robot Arm/DC Motors/Bicep Motor2/Power Amplifier/SL2Vbrk ==
  Signal : Inport
  Electrical Reference1 : fl_lib/Electrical/Electrical Elements/Electrical Reference
      settings: SourceProductBaseCode=MT,SS
  Simulink to Physical Signal1 : nesl_utility/Simulink-PS Converter  PhysicalDomain=network_engine_domain  SubClassName=ps_input  LeftPortType=input  RightPortType=output  PseudoPeriodic=off  Frequencies=[]  NoiseDistribution=none  NoiseParameters=[]  Unit=V  AffineConversion=off  FilteringAndDerivatives=zero  SimscapeFilterOrder=1  InputFilterTimeConstant=.001  UdotUserProvided=0
      settings: SourceProductBaseCode=MT,SS
  Voltage Source : fl_lib/Electrical/Electrical Sources/Controlled Voltage Source
      settings: SourceProductBaseCode=MT,SS
  Volts : PMIOPort  Tag=PMCPort  Side=Right
  wires:
  Signal/1 -> Simulink to Physical Signal1/1
  connections:
  Voltage Source/LConn1 -- Volts/RConn1
  Simulink to Physical Signal1/RConn1 -- Voltage Source/RConn1
  Electrical Reference1/LConn1 -- Voltage Source/RConn2

== system cst_robotarm_breach/6 DOF Robot Arm/DC Motors/Bicep Motor2/Power Amplifier/SL2Vduty ==
  Signal : Inport
  Electrical Reference1 : fl_lib/Electrical/Electrical Elements/Electrical Reference
      settings: SourceProductBaseCode=MT,SS
  Simulink to Physical Signal1 : nesl_utility/Simulink-PS Converter  PhysicalDomain=network_engine_domain  SubClassName=ps_input  LeftPortType=input  RightPortType=output  PseudoPeriodic=off  Frequencies=[]  NoiseDistribution=none  NoiseParameters=[]  Unit=V  AffineConversion=off  FilteringAndDerivatives=zero  SimscapeFilterOrder=1  InputFilterTimeConstant=.001  UdotUserProvided=0
      settings: SourceProductBaseCode=MT,SS
  Voltage Source : fl_lib/Electrical/Electrical Sources/Controlled Voltage Source
      settings: SourceProductBaseCode=MT,SS
  Volts : PMIOPort  Tag=PMCPort  Side=Right
  wires:
  Signal/1 -> Simulink to Physical Signal1/1
  connections:
  Voltage Source/LConn1 -- Volts/RConn1
  Simulink to Physical Signal1/RConn1 -- Voltage Source/RConn1
  Electrical Reference1/LConn1 -- Voltage Source/RConn2

== system cst_robotarm_breach/6 DOF Robot Arm/DC Motors/Bicep Motor2/Power Amplifier/SL2Vrev ==
  Signal : Inport
  Electrical Reference1 : fl_lib/Electrical/Electrical Elements/Electrical Reference
      settings: SourceProductBaseCode=MT,SS
  Simulink to Physical Signal1 : nesl_utility/Simulink-PS Converter  PhysicalDomain=network_engine_domain  SubClassName=ps_input  LeftPortType=input  RightPortType=output  PseudoPeriodic=off  Frequencies=[]  NoiseDistribution=none  NoiseParameters=[]  Unit=V  AffineConversion=off  FilteringAndDerivatives=zero  SimscapeFilterOrder=1  InputFilterTimeConstant=.001  UdotUserProvided=0
      settings: SourceProductBaseCode=MT,SS
  Voltage Source : fl_lib/Electrical/Electrical Sources/Controlled Voltage Source
      settings: SourceProductBaseCode=MT,SS
  Volts : PMIOPort  Tag=PMCPort  Side=Right
  wires:
  Signal/1 -> Simulink to Physical Signal1/1
  connections:
  Electrical Reference1/LConn1 -- Voltage Source/RConn2
  Simulink to Physical Signal1/RConn1 -- Voltage Source/RConn1
  Voltage Source/LConn1 -- Volts/RConn1

== system cst_robotarm_breach/6 DOF Robot Arm/DC Motors/Forearm Motor/Power Amplifier/SL2Vbrk ==
  Signal : Inport
  Electrical Reference1 : fl_lib/Electrical/Electrical Elements/Electrical Reference
      settings: SourceProductBaseCode=MT,SS
  Simulink to Physical Signal1 : nesl_utility/Simulink-PS Converter  PhysicalDomain=network_engine_domain  SubClassName=ps_input  LeftPortType=input  RightPortType=output  PseudoPeriodic=off  Frequencies=[]  NoiseDistribution=none  NoiseParameters=[]  Unit=V  AffineConversion=off  FilteringAndDerivatives=zero  SimscapeFilterOrder=1  InputFilterTimeConstant=.001  UdotUserProvided=0
      settings: SourceProductBaseCode=MT,SS
  Voltage Source : fl_lib/Electrical/Electrical Sources/Controlled Voltage Source
      settings: SourceProductBaseCode=MT,SS
  Volts : PMIOPort  Tag=PMCPort  Side=Right
  wires:
  Signal/1 -> Simulink to Physical Signal1/1
  connections:
  Voltage Source/LConn1 -- Volts/RConn1
  Simulink to Physical Signal1/RConn1 -- Voltage Source/RConn1
  Electrical Reference1/LConn1 -- Voltage Source/RConn2

== system cst_robotarm_breach/6 DOF Robot Arm/DC Motors/Forearm Motor/Power Amplifier/SL2Vduty ==
  Signal : Inport
  Electrical Reference1 : fl_lib/Electrical/Electrical Elements/Electrical Reference
      settings: SourceProductBaseCode=MT,SS
  Simulink to Physical Signal1 : nesl_utility/Simulink-PS Converter  PhysicalDomain=network_engine_domain  SubClassName=ps_input  LeftPortType=input  RightPortType=output  PseudoPeriodic=off  Frequencies=[]  NoiseDistribution=none  NoiseParameters=[]  Unit=V  AffineConversion=off  FilteringAndDerivatives=zero  SimscapeFilterOrder=1  InputFilterTimeConstant=.001  UdotUserProvided=0
      settings: SourceProductBaseCode=MT,SS
  Voltage Source : fl_lib/Electrical/Electrical Sources/Controlled Voltage Source
      settings: SourceProductBaseCode=MT,SS
  Volts : PMIOPort  Tag=PMCPort  Side=Right
  wires:
  Signal/1 -> Simulink to Physical Signal1/1
  connections:
  Voltage Source/LConn1 -- Volts/RConn1
  Simulink to Physical Signal1/RConn1 -- Voltage Source/RConn1
  Electrical Reference1/LConn1 -- Voltage Source/RConn2

== system cst_robotarm_breach/6 DOF Robot Arm/DC Motors/Forearm Motor/Power Amplifier/SL2Vrev ==
  Signal : Inport
  Electrical Reference1 : fl_lib/Electrical/Electrical Elements/Electrical Reference
      settings: SourceProductBaseCode=MT,SS
  Simulink to Physical Signal1 : nesl_utility/Simulink-PS Converter  PhysicalDomain=network_engine_domain  SubClassName=ps_input  LeftPortType=input  RightPortType=output  PseudoPeriodic=off  Frequencies=[]  NoiseDistribution=none  NoiseParameters=[]  Unit=V  AffineConversion=off  FilteringAndDerivatives=zero  SimscapeFilterOrder=1  InputFilterTimeConstant=.001  UdotUserProvided=0
      settings: SourceProductBaseCode=MT,SS
  Voltage Source : fl_lib/Electrical/Electrical Sources/Controlled Voltage Source
      settings: SourceProductBaseCode=MT,SS
  Volts : PMIOPort  Tag=PMCPort  Side=Right
  wires:
  Signal/1 -> Simulink to Physical Signal1/1
  connections:
  Electrical Reference1/LConn1 -- Voltage Source/RConn2
  Simulink to Physical Signal1/RConn1 -- Voltage Source/RConn1
  Voltage Source/LConn1 -- Volts/RConn1

== system cst_robotarm_breach/6 DOF Robot Arm/DC Motors/Hand Motor/Power Amplifier/SL2Vbrk ==
  Signal : Inport
  Electrical Reference1 : fl_lib/Electrical/Electrical Elements/Electrical Reference
      settings: SourceProductBaseCode=MT,SS
  Simulink to Physical Signal1 : nesl_utility/Simulink-PS Converter  PhysicalDomain=network_engine_domain  SubClassName=ps_input  LeftPortType=input  RightPortType=output  PseudoPeriodic=off  Frequencies=[]  NoiseDistribution=none  NoiseParameters=[]  Unit=V  AffineConversion=off  FilteringAndDerivatives=zero  SimscapeFilterOrder=1  InputFilterTimeConstant=.001  UdotUserProvided=0
      settings: SourceProductBaseCode=MT,SS
  Voltage Source : fl_lib/Electrical/Electrical Sources/Controlled Voltage Source
      settings: SourceProductBaseCode=MT,SS
  Volts : PMIOPort  Tag=PMCPort  Side=Right
  wires:
  Signal/1 -> Simulink to Physical Signal1/1
  connections:
  Voltage Source/LConn1 -- Volts/RConn1
  Simulink to Physical Signal1/RConn1 -- Voltage Source/RConn1
  Electrical Reference1/LConn1 -- Voltage Source/RConn2

== system cst_robotarm_breach/6 DOF Robot Arm/DC Motors/Hand Motor/Power Amplifier/SL2Vduty ==
  Signal : Inport
  Electrical Reference1 : fl_lib/Electrical/Electrical Elements/Electrical Reference
      settings: SourceProductBaseCode=MT,SS
  Simulink to Physical Signal1 : nesl_utility/Simulink-PS Converter  PhysicalDomain=network_engine_domain  SubClassName=ps_input  LeftPortType=input  RightPortType=output  PseudoPeriodic=off  Frequencies=[]  NoiseDistribution=none  NoiseParameters=[]  Unit=V  AffineConversion=off  FilteringAndDerivatives=zero  SimscapeFilterOrder=1  InputFilterTimeConstant=.001  UdotUserProvided=0
      settings: SourceProductBaseCode=MT,SS
  Voltage Source : fl_lib/Electrical/Electrical Sources/Controlled Voltage Source
      settings: SourceProductBaseCode=MT,SS
  Volts : PMIOPort  Tag=PMCPort  Side=Right
  wires:
  Signal/1 -> Simulink to Physical Signal1/1
  connections:
  Voltage Source/LConn1 -- Volts/RConn1
  Simulink to Physical Signal1/RConn1 -- Voltage Source/RConn1
  Electrical Reference1/LConn1 -- Voltage Source/RConn2

== system cst_robotarm_breach/6 DOF Robot Arm/DC Motors/Hand Motor/Power Amplifier/SL2Vrev ==
  Signal : Inport
  Electrical Reference1 : fl_lib/Electrical/Electrical Elements/Electrical Reference
      settings: SourceProductBaseCode=MT,SS
  Simulink to Physical Signal1 : nesl_utility/Simulink-PS Converter  PhysicalDomain=network_engine_domain  SubClassName=ps_input  LeftPortType=input  RightPortType=output  PseudoPeriodic=off  Frequencies=[]  NoiseDistribution=none  NoiseParameters=[]  Unit=V  AffineConversion=off  FilteringAndDerivatives=zero  SimscapeFilterOrder=1  InputFilterTimeConstant=.001  UdotUserProvided=0
      settings: SourceProductBaseCode=MT,SS
  Voltage Source : fl_lib/Electrical/Electrical Sources/Controlled Voltage Source
      settings: SourceProductBaseCode=MT,SS
  Volts : PMIOPort  Tag=PMCPort  Side=Right
  wires:
  Signal/1 -> Simulink to Physical Signal1/1
  connections:
  Electrical Reference1/LConn1 -- Voltage Source/RConn2
  Simulink to Physical Signal1/RConn1 -- Voltage Source/RConn1
  Voltage Source/LConn1 -- Volts/RConn1

== system cst_robotarm_breach/6 DOF Robot Arm/DC Motors/Hand Motor1/Power Amplifier/SL2Vbrk ==
  Signal : Inport
  Electrical Reference1 : fl_lib/Electrical/Electrical Elements/Electrical Reference
      settings: SourceProductBaseCode=MT,SS
  Simulink to Physical Signal1 : nesl_utility/Simulink-PS Converter  PhysicalDomain=network_engine_domain  SubClassName=ps_input  LeftPortType=input  RightPortType=output  PseudoPeriodic=off  Frequencies=[]  NoiseDistribution=none  NoiseParameters=[]  Unit=V  AffineConversion=off  FilteringAndDerivatives=zero  SimscapeFilterOrder=1  InputFilterTimeConstant=.001  UdotUserProvided=0
      settings: SourceProductBaseCode=MT,SS
  Voltage Source : fl_lib/Electrical/Electrical Sources/Controlled Voltage Source
      settings: SourceProductBaseCode=MT,SS
  Volts : PMIOPort  Tag=PMCPort  Side=Right
  wires:
  Signal/1 -> Simulink to Physical Signal1/1
  connections:
  Electrical Reference1/LConn1 -- Voltage Source/RConn2
  Simulink to Physical Signal1/RConn1 -- Voltage Source/RConn1
  Voltage Source/LConn1 -- Volts/RConn1

== system cst_robotarm_breach/6 DOF Robot Arm/DC Motors/Hand Motor1/Power Amplifier/SL2Vduty ==
  Signal : Inport
  Electrical Reference1 : fl_lib/Electrical/Electrical Elements/Electrical Reference
      settings: SourceProductBaseCode=MT,SS
  Simulink to Physical Signal1 : nesl_utility/Simulink-PS Converter  PhysicalDomain=network_engine_domain  SubClassName=ps_input  LeftPortType=input  RightPortType=output  PseudoPeriodic=off  Frequencies=[]  NoiseDistribution=none  NoiseParameters=[]  Unit=V  AffineConversion=off  FilteringAndDerivatives=zero  SimscapeFilterOrder=1  InputFilterTimeConstant=.001  UdotUserProvided=0
      settings: SourceProductBaseCode=MT,SS
  Voltage Source : fl_lib/Electrical/Electrical Sources/Controlled Voltage Source
      settings: SourceProductBaseCode=MT,SS
  Volts : PMIOPort  Tag=PMCPort  Side=Right
  wires:
  Signal/1 -> Simulink to Physical Signal1/1
  connections:
  Electrical Reference1/LConn1 -- Voltage Source/RConn2
  Simulink to Physical Signal1/RConn1 -- Voltage Source/RConn1
  Voltage Source/LConn1 -- Volts/RConn1
